simulink model "Transitions5"  (R2020a)
settings: Solver=VariableStepAuto  StartTime=0.0  StopTime=0.1  RelTol=1e-3
settings Model: Creator=BEAR  LastModifiedBy=bzhan
settings DataIOCC: ReturnWorkspaceOutputs=off
settings DebuggingCC: ArithmeticOperatorsInVariantConditions=warning
settings SFSimCC: SimUseLocalCustomCode=off  CustomCodeUndefinedFunction=UseInterfaceOnly
settings RTWCC: RTWUseLocalCustomCode=off

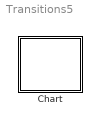
== system Transitions5 ==
  Chart : Stateflow chart  TreatAsAtomicUnit=on

== stateflow chart Transitions5/Chart ==
  settings: updateMethod=DISCRETE  sampleTime=0.1
  state S
    en: f("enS")
    du: f("duS")
    state A
      en: f("enA")
      ex: f("exA")
    state B
      en: f("enB")
      ex: f("exB")
    S -> S : {f("condInner")}/{f("tranInner")}
    (default) -> A
    A -> B
    B -> A
  (default) -> S
  data: s function_input
  function f(s):
    | function f(s)
    |   fprintf(s+"\n");
